simulink model "fermentationModel"  (R2014a)
settings: Solver=ode45  StartTime=0.0  StopTime=10.0  RelTol=1e-3
InitFcn:
  | initParams();
values from neighbouring files (symbols this model uses):
  E_G0 = 22.6    [initParams.m]
  E_KG = -68.6    [initParams.m]
  E_KM = -14.4    [initParams.m]
  E_KN = -19.9    [initParams.m]
  E_M0 = 11.3    [initParams.m]
  E_N0 = 7.16    [initParams.m]
  Ed_G0 = exp(23.33)    [initParams.m]
  Ed_KG = 10.2    [initParams.m]
  Ed_KM = 26.3    [initParams.m]
  Ed_M0 = exp(55.61)    [initParams.m]
  G0 = 1    [initParams.m]
  K_G0 = exp(-121.3)    [initParams.m]
  K_M0 = exp(-19.5)    [initParams.m]
  K_N0 = exp(-26.78)    [initParams.m]
  Kx = 365000    [initParams.m]
  M0 = 1    [initParams.m]
  mu_G0 = exp(35.77)    [initParams.m]
  mu_M0 = exp(16.4)    [initParams.m]
  mu_N0 = exp(10.59)    [initParams.m]
  N0 = 1    [initParams.m]
  R = 1.9872041e-3    (= 0.0019872041)    [initParams.m]
  X0 = 1    [initParams.m]
  Y_XG = 0.134    [initParams.m]
  Y_XM = -0.268    [initParams.m]
  Y_XN = 0.402    [initParams.m]
settings Model: Creator=jlesage  LastModifiedBy=jlesage

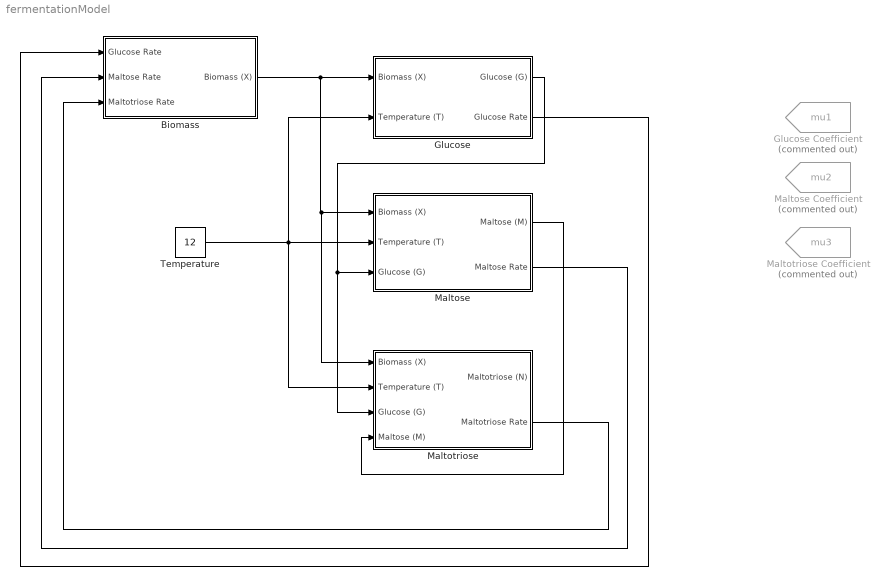
== system fermentationModel ==
  Biomass : Subsystem
  Glucose : Subsystem
  Glucose Coefficient : Goto  Commented=on  GotoTag=mu1  TagVisibility=global
  Maltose : Subsystem
  Maltose Coefficient : Goto  Commented=on  GotoTag=mu2  TagVisibility=global
  Maltotriose : Subsystem
  Maltotriose Coefficient : Goto  Commented=on  GotoTag=mu3  TagVisibility=global
  Temperature : Constant  Value=12
  wires:
  Biomass/1(Biomass (X)) -> Maltotriose/1(Biomass (X)), Maltose/1(Biomass (X)), Glucose/1(Biomass (X))
  Glucose/2(Glucose Rate) -> Biomass/1(Glucose Rate)
  Maltose/2(Maltose Rate) -> Biomass/2(Maltose Rate)
  Maltotriose/2(Maltotriose Rate) -> Biomass/3(Maltotriose Rate)
  Glucose/1(Glucose (G)) -> Maltose/3(Glucose (G)), Maltotriose/3(Glucose (G))
  Maltose/1(Maltose (M)) -> Maltotriose/4(Maltose (M))
  Temperature/1 -> Maltotriose/2(Temperature (T)), Maltose/2(Temperature (T)), Glucose/2(Temperature (T))

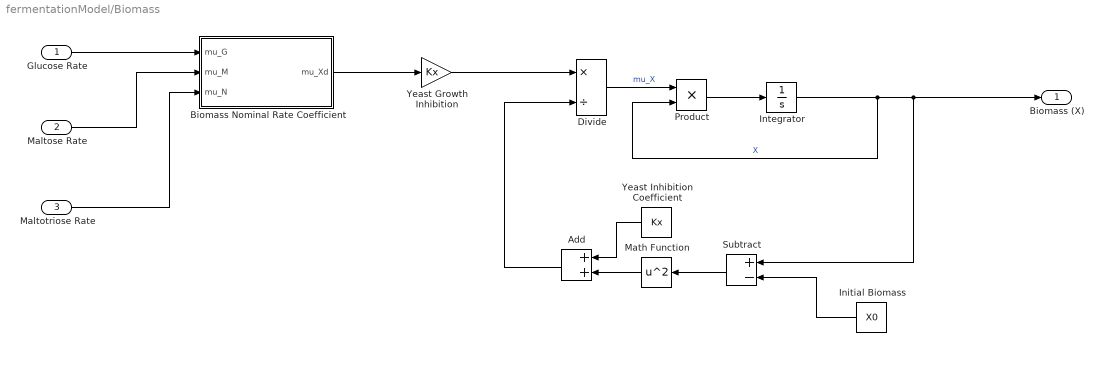
== system fermentationModel/Biomass ==
  Glucose Rate : Inport
  Maltose Rate : Inport  Port=2
  Maltotriose Rate : Inport  Port=3
  Add : Sum
  Biomass Nominal Rate Coefficient : Subsystem
  Divide : Product  Inputs=*/
  Initial Biomass : Constant  Value=X0
  Integrator : Integrator  InitialCondition=X0
  Math Function : Math  Operator=square  SaturateOnIntegerOverflow=on
  Product : Product
  Subtract : Sum  Inputs=+-
  Yeast Growth Inhibition : Gain  Gain=Kx
  Yeast Inhibition Coefficient : Constant  Value=Kx
  Biomass (X) : Outport
  wires:
  Glucose Rate/1 -> Biomass Nominal Rate Coefficient/1(mu_G)
  Maltose Rate/1 -> Biomass Nominal Rate Coefficient/2(mu_M)
  Maltotriose Rate/1 -> Biomass Nominal Rate Coefficient/3(mu_N)
  Integrator/1 -> Product/2, Subtract/1, Biomass (X)/1  "X"
  Biomass Nominal Rate Coefficient/1(mu_Xd) -> Yeast Growth Inhibition/1
  Yeast Growth Inhibition/1 -> Divide/1
  Initial Biomass/1 -> Subtract/2
  Subtract/1 -> Math Function/1
  Math Function/1 -> Add/2
  Yeast Inhibition Coefficient/1 -> Add/1
  Add/1 -> Divide/2
  Divide/1 -> Product/1  "mu_X"
  Product/1 -> Integrator/1

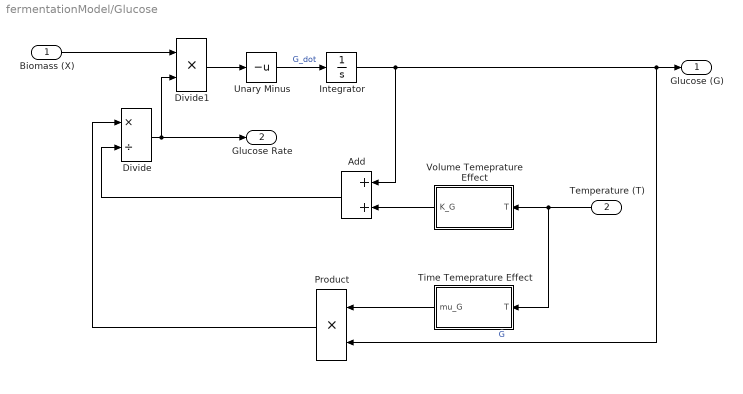
== system fermentationModel/Glucose ==
  Biomass (X) : Inport
  Temperature (T) : Inport  Port=2
  Add : Sum
  Divide : Product  Inputs=*/
  Divide1 : Product  Inputs=**
  Integrator : Integrator  InitialCondition=G0
  Product : Product
  Time Temeprature Effect : Subsystem
  Unary Minus : UnaryMinus
  Volume Temeprature Effect : Subsystem
  Glucose (G) : Outport
  Glucose Rate : Outport  Port=2
  wires:
  Temperature (T)/1 -> Time Temeprature Effect/1(T), Volume Temeprature Effect/1(T)
  Integrator/1 -> Add/1, Product/2, Glucose (G)/1  "G"
  Volume Temeprature Effect/1(K_G) -> Add/2
  Unary Minus/1 -> Integrator/1  "G_dot"
  Product/1 -> Divide/1
  Add/1 -> Divide/2
  Time Temeprature Effect/1(mu_G) -> Product/1
  Divide/1 -> Glucose Rate/1, Divide1/2
  Biomass (X)/1 -> Divide1/1
  Divide1/1 -> Unary Minus/1

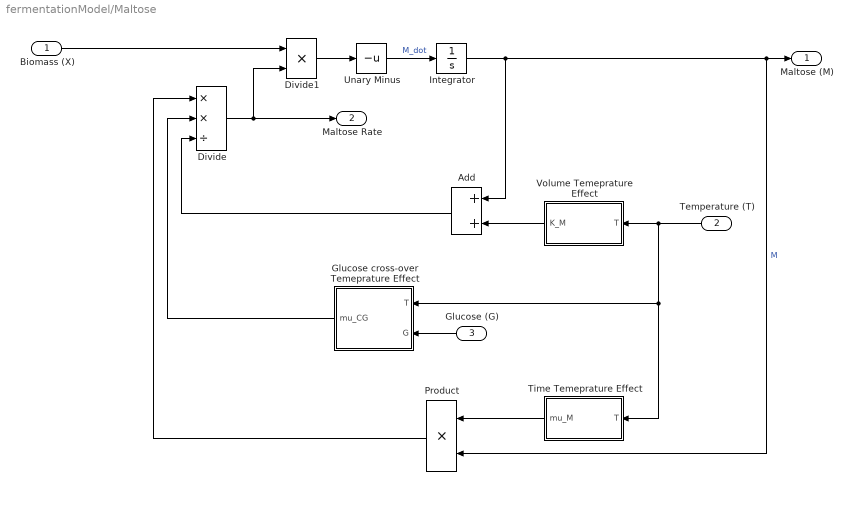
== system fermentationModel/Maltose ==
  Biomass (X) : Inport
  Temperature (T) : Inport  Port=2
  Glucose (G) : Inport  Port=3
  Add : Sum
  Divide : Product  Inputs=**/
  Divide1 : Product  Inputs=**
  Glucose cross-over Temeprature Effect : Subsystem
  Integrator : Integrator  InitialCondition=M0
  Product : Product
  Time Temeprature Effect : Subsystem
  Unary Minus : UnaryMinus
  Volume Temeprature Effect : Subsystem
  Maltose (M) : Outport
  Maltose Rate : Outport  Port=2
  wires:
  Time Temeprature Effect/1(mu_M) -> Product/1
  Add/1 -> Divide/3
  Product/1 -> Divide/1
  Biomass (X)/1 -> Divide1/1
  Unary Minus/1 -> Integrator/1  "M_dot"
  Divide/1 -> Maltose Rate/1, Divide1/2
  Volume Temeprature Effect/1(K_M) -> Add/2
  Integrator/1 -> Add/1, Product/2, Maltose (M)/1  "M"
  Temperature (T)/1 -> Volume Temeprature Effect/1(T), Time Temeprature Effect/1(T), Glucose cross-over Temeprature Effect/1(T)
  Glucose cross-over Temeprature Effect/1(mu_CG) -> Divide/2
  Glucose (G)/1 -> Glucose cross-over Temeprature Effect/2(G)
  Divide1/1 -> Unary Minus/1

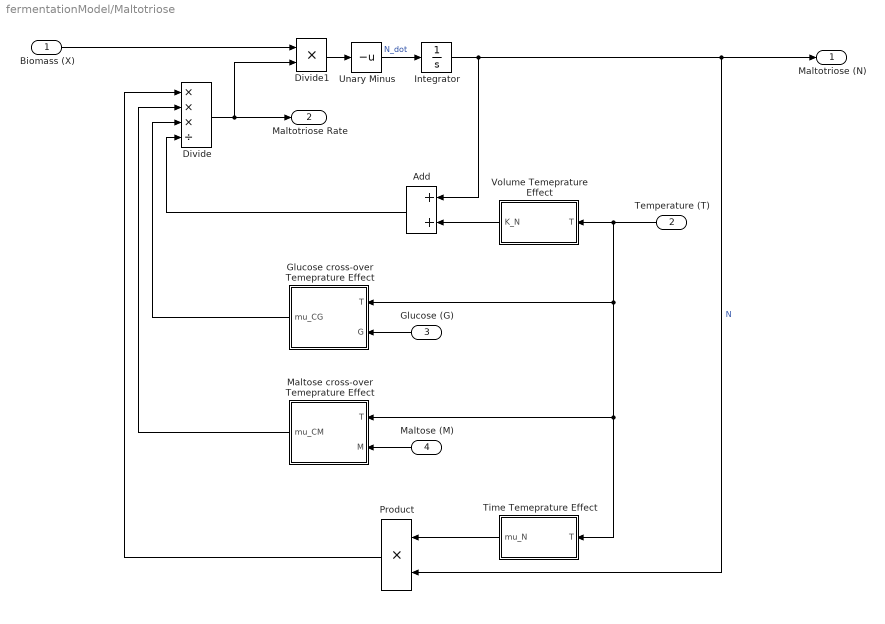
== system fermentationModel/Maltotriose ==
  Biomass (X) : Inport
  Temperature (T) : Inport  Port=2
  Glucose (G) : Inport  Port=3
  Maltose (M) : Inport  Port=4
  Add : Sum
  Divide : Product  Inputs=***/
  Divide1 : Product  Inputs=**
  Glucose cross-over Temeprature Effect : Subsystem
  Integrator : Integrator  InitialCondition=N0
  Maltose cross-over Temeprature Effect : Subsystem
  Product : Product
  Time Temeprature Effect : Subsystem
  Unary Minus : UnaryMinus
  Volume Temeprature Effect : Subsystem
  Maltotriose (N) : Outport
  Maltotriose Rate : Outport  Port=2
  wires:
  Glucose (G)/1 -> Glucose cross-over Temeprature Effect/2(G)
  Glucose cross-over Temeprature Effect/1(mu_CG) -> Divide/3
  Temperature (T)/1 -> Glucose cross-over Temeprature Effect/1(T), Maltose cross-over Temeprature Effect/1(T), Time Temeprature Effect/1(T), Volume Temeprature Effect/1(T)
  Integrator/1 -> Add/1, Product/2, Maltotriose (N)/1  "N"
  Volume Temeprature Effect/1(K_N) -> Add/2
  Unary Minus/1 -> Integrator/1  "N_dot"
  Biomass (X)/1 -> Divide1/1
  Product/1 -> Divide/1
  Add/1 -> Divide/4
  Time Temeprature Effect/1(mu_N) -> Product/1
  Maltose (M)/1 -> Maltose cross-over Temeprature Effect/2(M)
  Maltose cross-over Temeprature Effect/1(mu_CM) -> Divide/2
  Divide/1 -> Maltotriose Rate/1, Divide1/2
  Divide1/1 -> Unary Minus/1

== system fermentationModel/Biomass/Biomass Nominal Rate Coefficient ==
  mu_G : Inport
  mu_M : Inport  Port=2
  mu_N : Inport  Port=3
  Add : Sum  Inputs=+++
  Glucose Yield Coefficient : Gain  Gain=Y_XG
  Maltose Yield Coefficient : Gain  Gain=Y_XM
  Maltotriose Yield Coefficient : Gain  Gain=Y_XN
  mu_Xd : Outport
  wires:
  Add/1 -> mu_Xd/1
  mu_G/1 -> Glucose Yield Coefficient/1
  mu_M/1 -> Maltose Yield Coefficient/1
  mu_N/1 -> Maltotriose Yield Coefficient/1
  Glucose Yield Coefficient/1 -> Add/1
  Maltose Yield Coefficient/1 -> Add/2
  Maltotriose Yield Coefficient/1 -> Add/3

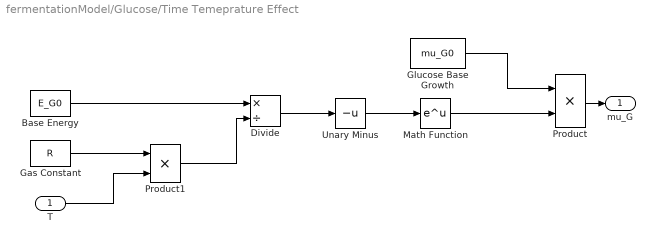
== system fermentationModel/Glucose/Time Temeprature Effect ==
  T : Inport
  Base Energy : Constant  Value=E_G0
  Divide : Product  Inputs=*/
  Gas Constant : Constant  Value=R
  Glucose Base Growth : Constant  Value=mu_G0
  Math Function : Math  SaturateOnIntegerOverflow=on
  Product : Product
  Product1 : Product
  Unary Minus : UnaryMinus
  mu_G : Outport
  wires:
  Product1/1 -> Divide/2
  Gas Constant/1 -> Product1/1
  Math Function/1 -> Product/2
  Base Energy/1 -> Divide/1
  Glucose Base Growth/1 -> Product/1
  T/1 -> Product1/2
  Divide/1 -> Unary Minus/1
  Unary Minus/1 -> Math Function/1
  Product/1 -> mu_G/1

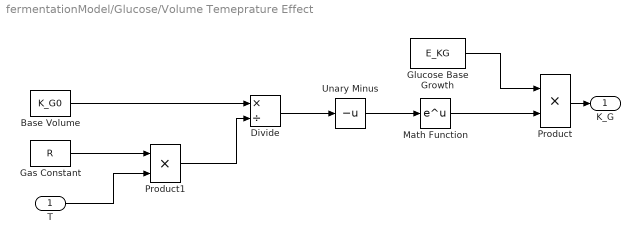
== system fermentationModel/Glucose/Volume Temeprature Effect ==
  T : Inport
  Base Volume : Constant  Value=K_G0
  Divide : Product  Inputs=*/
  Gas Constant : Constant  Value=R
  Glucose Base Growth : Constant  Value=E_KG
  Math Function : Math  SaturateOnIntegerOverflow=on
  Product : Product
  Product1 : Product
  Unary Minus : UnaryMinus
  K_G : Outport
  wires:
  Product/1 -> K_G/1
  Unary Minus/1 -> Math Function/1
  Divide/1 -> Unary Minus/1
  T/1 -> Product1/2
  Glucose Base Growth/1 -> Product/1
  Base Volume/1 -> Divide/1
  Math Function/1 -> Product/2
  Gas Constant/1 -> Product1/1
  Product1/1 -> Divide/2

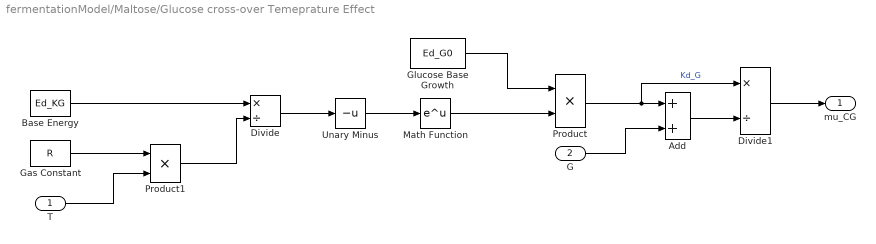
== system fermentationModel/Maltose/Glucose cross-over Temeprature Effect ==
  T : Inport
  G : Inport  Port=2
  Add : Sum
  Base Energy : Constant  Value=Ed_KG
  Divide : Product  Inputs=*/
  Divide1 : Product  Inputs=*/
  Gas Constant : Constant  Value=R
  Glucose Base Growth : Constant  Value=Ed_G0
  Math Function : Math  SaturateOnIntegerOverflow=on
  Product : Product
  Product1 : Product
  Unary Minus : UnaryMinus
  mu_CG : Outport
  wires:
  Product1/1 -> Divide/2
  Gas Constant/1 -> Product1/1
  Math Function/1 -> Product/2
  Base Energy/1 -> Divide/1
  Glucose Base Growth/1 -> Product/1
  T/1 -> Product1/2
  Divide/1 -> Unary Minus/1
  Unary Minus/1 -> Math Function/1
  Product/1 -> Divide1/1, Add/1  "Kd_G"
  G/1 -> Add/2
  Add/1 -> Divide1/2
  Divide1/1 -> mu_CG/1

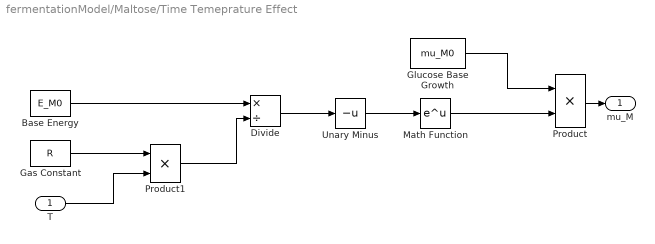
== system fermentationModel/Maltose/Time Temeprature Effect ==
  T : Inport
  Base Energy : Constant  Value=E_M0
  Divide : Product  Inputs=*/
  Gas Constant : Constant  Value=R
  Glucose Base Growth : Constant  Value=mu_M0
  Math Function : Math  SaturateOnIntegerOverflow=on
  Product : Product
  Product1 : Product
  Unary Minus : UnaryMinus
  mu_M : Outport
  wires:
  Product/1 -> mu_M/1
  Unary Minus/1 -> Math Function/1
  Divide/1 -> Unary Minus/1
  T/1 -> Product1/2
  Glucose Base Growth/1 -> Product/1
  Base Energy/1 -> Divide/1
  Math Function/1 -> Product/2
  Gas Constant/1 -> Product1/1
  Product1/1 -> Divide/2

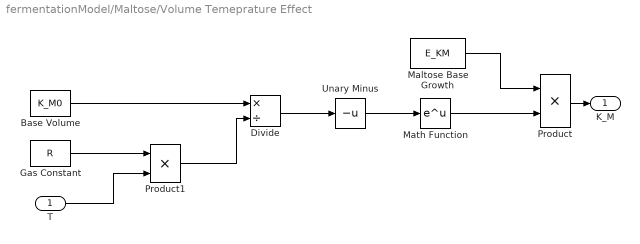
== system fermentationModel/Maltose/Volume Temeprature Effect ==
  T : Inport
  Base Volume : Constant  Value=K_M0
  Divide : Product  Inputs=*/
  Gas Constant : Constant  Value=R
  Maltose Base Growth : Constant  Value=E_KM
  Math Function : Math  SaturateOnIntegerOverflow=on
  Product : Product
  Product1 : Product
  Unary Minus : UnaryMinus
  K_M : Outport
  wires:
  Product1/1 -> Divide/2
  Gas Constant/1 -> Product1/1
  Math Function/1 -> Product/2
  Base Volume/1 -> Divide/1
  Maltose Base Growth/1 -> Product/1
  T/1 -> Product1/2
  Divide/1 -> Unary Minus/1
  Unary Minus/1 -> Math Function/1
  Product/1 -> K_M/1

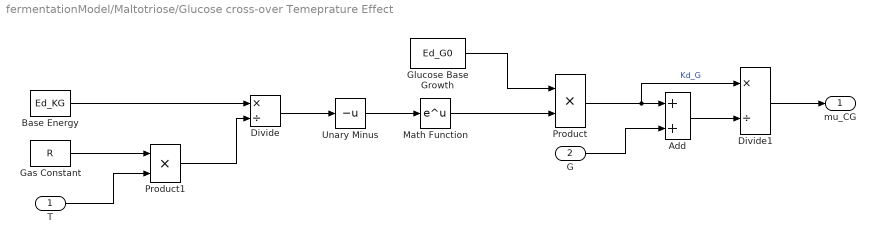
== system fermentationModel/Maltotriose/Glucose cross-over Temeprature Effect ==
  T : Inport
  G : Inport  Port=2
  Add : Sum
  Base Energy : Constant  Value=Ed_KG
  Divide : Product  Inputs=*/
  Divide1 : Product  Inputs=*/
  Gas Constant : Constant  Value=R
  Glucose Base Growth : Constant  Value=Ed_G0
  Math Function : Math  SaturateOnIntegerOverflow=on
  Product : Product
  Product1 : Product
  Unary Minus : UnaryMinus
  mu_CG : Outport
  wires:
  Divide1/1 -> mu_CG/1
  Add/1 -> Divide1/2
  G/1 -> Add/2
  Product/1 -> Add/1, Divide1/1  "Kd_G"
  Unary Minus/1 -> Math Function/1
  Divide/1 -> Unary Minus/1
  T/1 -> Product1/2
  Glucose Base Growth/1 -> Product/1
  Base Energy/1 -> Divide/1
  Math Function/1 -> Product/2
  Gas Constant/1 -> Product1/1
  Product1/1 -> Divide/2

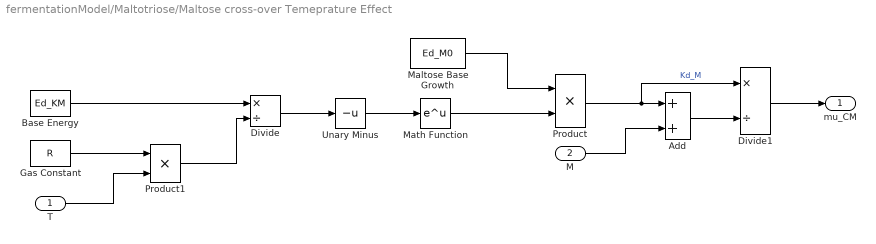
== system fermentationModel/Maltotriose/Maltose cross-over Temeprature Effect ==
  T : Inport
  M : Inport  Port=2
  Add : Sum
  Base Energy : Constant  Value=Ed_KM
  Divide : Product  Inputs=*/
  Divide1 : Product  Inputs=*/
  Gas Constant : Constant  Value=R
  Maltose Base Growth : Constant  Value=Ed_M0
  Math Function : Math  SaturateOnIntegerOverflow=on
  Product : Product
  Product1 : Product
  Unary Minus : UnaryMinus
  mu_CM : Outport
  wires:
  Product1/1 -> Divide/2
  Gas Constant/1 -> Product1/1
  Math Function/1 -> Product/2
  Base Energy/1 -> Divide/1
  Maltose Base Growth/1 -> Product/1
  T/1 -> Product1/2
  Divide/1 -> Unary Minus/1
  Unary Minus/1 -> Math Function/1
  Product/1 -> Divide1/1, Add/1  "Kd_M"
  M/1 -> Add/2
  Add/1 -> Divide1/2
  Divide1/1 -> mu_CM/1

== system fermentationModel/Maltotriose/Time Temeprature Effect ==
  T : Inport
  Base Energy : Constant  Value=E_N0
  Divide : Product  Inputs=*/
  Gas Constant : Constant  Value=R
  Maltotriose Base Growth : Constant  Value=mu_N0
  Math Function : Math  SaturateOnIntegerOverflow=on
  Product : Product
  Product1 : Product
  Unary Minus : UnaryMinus
  mu_N : Outport
  wires:
  Product1/1 -> Divide/2
  Gas Constant/1 -> Product1/1
  Math Function/1 -> Product/2
  Base Energy/1 -> Divide/1
  Maltotriose Base Growth/1 -> Product/1
  T/1 -> Product1/2
  Divide/1 -> Unary Minus/1
  Unary Minus/1 -> Math Function/1
  Product/1 -> mu_N/1

== system fermentationModel/Maltotriose/Volume Temeprature Effect ==
  T : Inport
  Base Volume : Constant  Value=K_N0
  Divide : Product  Inputs=*/
  Gas Constant : Constant  Value=R
  Maltotriose Base Growth : Constant  Value=E_KN
  Math Function : Math  SaturateOnIntegerOverflow=on
  Product : Product
  Product1 : Product
  Unary Minus : UnaryMinus
  K_N : Outport
  wires:
  Product/1 -> K_N/1
  Unary Minus/1 -> Math Function/1
  Divide/1 -> Unary Minus/1
  T/1 -> Product1/2
  Maltotriose Base Growth/1 -> Product/1
  Base Volume/1 -> Divide/1
  Math Function/1 -> Product/2
  Gas Constant/1 -> Product1/1
  Product1/1 -> Divide/2
